simulink model "sim_instalacja_grzejnikowa_modele"  (R2021b)
settings: Solver=VariableStepAuto  StartTime=0.0  StopTime=10.0  MaxStep=1  RelTol=1e-3
undefined symbols (not defined in the file): dspr, k, skok_czas, T0_klasyczna, T_klasyczna
settings Model: Creator=adams  LastModifiedBy=adams

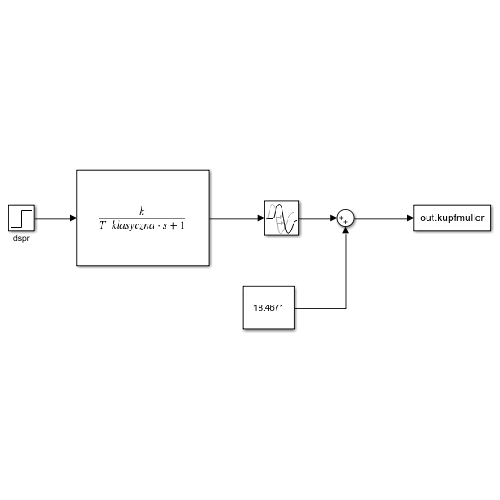
[thumbnail: Simulink's stored preview of the top-level diagram]
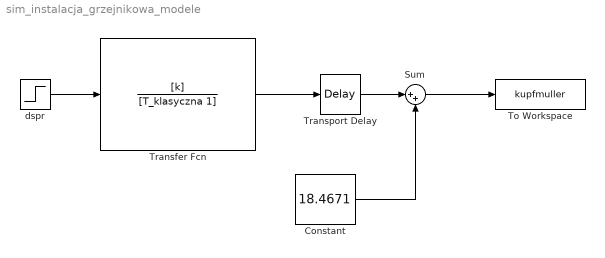
== system sim_instalacja_grzejnikowa_modele ==
  Constant : Constant  Value=18.4671
  Sum : Sum  Inputs=|++
  To Workspace : ToWorkspace  VariableName=kupfmuller  SampleTime=-1
  Transfer Fcn : TransferFcn  Numerator=[k]  Denominator=[T_klasyczna 1]
  Transport Delay : TransportDelay  DelayTime=T0_klasyczna  BufferSize=32768
  dspr : Step  Time=skok_czas  After=dspr  SampleTime=0
  wires:
  Sum/1 -> To Workspace/1
  Constant/1 -> Sum/2
  Transport Delay/1 -> Sum/1
  Transfer Fcn/1 -> Transport Delay/1
  dspr/1 -> Transfer Fcn/1
